simulink model "gm_VSD_and_Park_transformation_6Phase"  (R2022a)
settings: Solver=FixedStepDiscrete  StartTime=0.0  StopTime=0.2  RelTol=1e-3
libraries: hdlmdlgenlib x2
(part 1 of 2)
settings Model: Creator=Andre Merx  LastModifiedBy=Andre Merx
settings SolverCC: AlgebraicLoopSolver=TrustRegion
settings DataIOCC: LimitDataPoints=on  SaveOutput=off  SaveTime=off
settings OptimizationCC: BlockReduction=off  ConditionallyExecuteInputs=off  DefaultParameterBehavior=Inlined  InheritOutputTypeSmallerThanSingle=on  LifeSpan=inf
settings DebuggingCC: AlgebraicLoopMsg=error  InheritedTsInSrcMsg=none  SingleTaskRateTransMsg=error  UnconnectedInputMsg=warning  UnconnectedOutputMsg=warning  UnconnectedLineMsg=warning  AllowSymbolicDim=off  StrictBusMsg=ErrorOnBusTreatedAsVector  SFUnexpectedBacktrackingDiag=warning  SFNoUnconditionalDefaultTransitionDiag=warning  SFExecutionAtInitializationDiag=none  SFMachineParentedDataDiag=warning  ArithmeticOperatorsInVariantConditions=warning
settings HardwareCC: ProdBitPerPointer=32  ProdBitPerSizeT=32  ProdBitPerPtrDiffT=32  ProdLargestAtomicFloat=None  ProdIntDivRoundTo=Undefined  ProdEndianess=Unspecified  ProdWordSize=32  ProdHWDeviceType=ASIC/FPGA->ASIC/FPGA  ProdEqTarget=off
settings SFSimCC: SimUseLocalCustomCode=off  CustomCodeUndefinedFunction=UseInterfaceOnly
settings RTWCC: RTWUseLocalCustomCode=off
settings CodeAppCC: StateflowObjectComments=on
settings GRTTargetCC: TargetLangStandard=C89/C90 (ANSI)
settings ConfigComp: CovScope=ReferencedModels  CovMetricSettings=dw  CovSaveCumulativeToWorkspaceVar=on  CovSaveSingleToWorkspaceVar=on  CovExternalEMLEnable=off  CovSFcnEnable=off

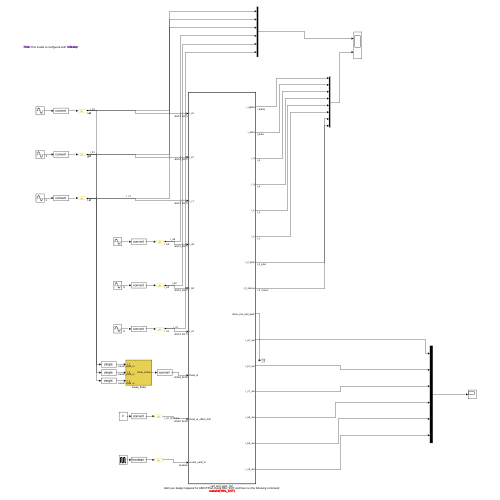
[thumbnail: Simulink's stored preview of the top-level diagram]
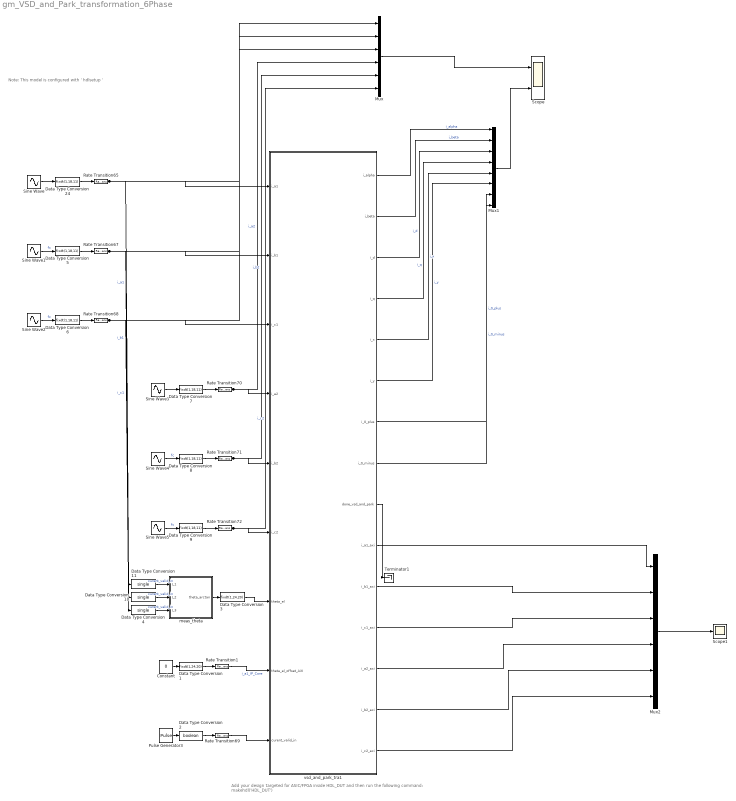
== system gm_VSD_and_Park_transformation_6Phase ==
  note: Add your design targeted for ASIC/FPGA inside HDL_DUT and then run the following command:
      | makehdl('HDL_DUT')
  note: Note: This model is configured with ' hdlsetup '
  Constant : Constant  Value=0  SampleTime=-1
  Data Type Conversion1 : DataTypeConversion  OutDataTypeStr=fixdt(1,24,20)  SaturateOnIntegerOverflow=off  RndMeth=Floor
  Data Type Conversion10 : DataTypeConversion  OutDataTypeStr=single  SaturateOnIntegerOverflow=off  RndMeth=Floor
  Data Type Conversion11 : DataTypeConversion  OutDataTypeStr=single  SaturateOnIntegerOverflow=off  RndMeth=Floor
  Data Type Conversion2 : DataTypeConversion  OutDataTypeStr=boolean  SaturateOnIntegerOverflow=off  RndMeth=Floor
  Data Type Conversion{5..9,24} (6 alike) : DataTypeConversion  OutDataTypeStr=fixdt(1,18,11)  SaturateOnIntegerOverflow=off  RndMeth=Floor
  Data Type Conversion3 : DataTypeConversion  OutDataTypeStr=fixdt(1,24,20)  SaturateOnIntegerOverflow=off  RndMeth=Floor
  Data Type Conversion4 : DataTypeConversion  OutDataTypeStr=single  SaturateOnIntegerOverflow=off  RndMeth=Floor
  Mux : Mux  Inputs=6
  Mux1 : Mux  Inputs=8
  Mux2 : Mux  Inputs=6
  Pulse Generator3 : DiscretePulseGenerator  PulseType=Time based  Period=1/100000  PulseWidth=5
  Rate Transition{1,65,67..72} (8 alike) : RateTransition  OutPortSampleTime=1.0000e-08
  Scope : Scope  NumInputPorts=2
  Scope1 : Scope
  Sine Wave : Sin  Frequency=100  SampleTime=1/100000
  Sine Wave1 : Sin  Frequency=100  Phase=(4/3)*pi  SampleTime=1/100000
  Sine Wave2 : Sin  Frequency=100  Phase=(2/3)*pi  SampleTime=1/100000
  Sine Wave3 : Sin  Amplitude=0.5  Frequency=100  Phase=-pi/6  SampleTime=1/100000
  Sine Wave4 : Sin  Amplitude=0.5  Frequency=100  Phase=(7/6)*pi  SampleTime=1/100000
  Sine Wave5 : Sin  Amplitude=0.5  Frequency=100  Phase=(1/2)*pi  SampleTime=1/100000
  Terminator1 : Terminator
  meas_theta : Subsystem
  vsd_and_park_tra1 : Subsystem  TreatAsAtomicUnit=on
  wires:
  vsd_and_park_tra1/6(i_y) -> Mux1/6  "i_y"
  vsd_and_park_tra1/7(i_0_plus) -> Mux1/7  "i_0_plus"
  vsd_and_park_tra1/8(i_0_minus) -> Mux1/8  "i_0_minus"
  vsd_and_park_tra1/9(done_vsd_and_park) -> Terminator1/1
  Mux2/1 -> Scope1/1
  vsd_and_park_tra1/15(i_c2_axi) -> Mux2/6
  vsd_and_park_tra1/14(i_b2_axi) -> Mux2/5
  vsd_and_park_tra1/13(i_a2_axi) -> Mux2/4
  vsd_and_park_tra1/12(i_c1_axi) -> Mux2/3
  vsd_and_park_tra1/11(i_b1_axi) -> Mux2/2
  vsd_and_park_tra1/10(i_a1_axi) -> Mux2/1
  Data Type Conversion11/1 -> meas_theta/1(I_1)  "curent_valid_in"
  Data Type Conversion10/1 -> meas_theta/2(I_2)  "curent_valid_in"
  Data Type Conversion4/1 -> meas_theta/3(I_3)  "curent_valid_in"
  Data Type Conversion3/1 -> vsd_and_park_tra1/7(theta_el)
  Mux1/1 -> Scope/2
  vsd_and_park_tra1/5(i_x) -> Mux1/5  "i_x"
  vsd_and_park_tra1/4(i_q) -> Mux1/4  "i_q"
  vsd_and_park_tra1/3(i_d) -> Mux1/3  "i_d"
  vsd_and_park_tra1/2(i_beta) -> Mux1/2  "i_beta"
  vsd_and_park_tra1/1(i_alpha) -> Mux1/1  "i_alpha"
  Mux/1 -> Scope/1
  Data Type Conversion2/1 -> Rate Transition69/1
  Rate Transition69/1 -> vsd_and_park_tra1/9(curent_valid_in)
  Pulse Generator3/1 -> Data Type Conversion2/1
  Rate Transition1/1 -> vsd_and_park_tra1/8(theta_el_offset_AXI)  "i_a1_IP_Core"
  Data Type Conversion1/1 -> Rate Transition1/1
  Constant/1 -> Data Type Conversion1/1
  meas_theta/1(theta_arctan) -> Data Type Conversion3/1
  Rate Transition72/1 -> Mux/6, vsd_and_park_tra1/6(i_c2)  "i_c2"
  Rate Transition71/1 -> Mux/5, vsd_and_park_tra1/5(i_b2)  "i_b2"
  Rate Transition70/1 -> Mux/4, vsd_and_park_tra1/4(i_a2)  "i_a2"
  Data Type Conversion8/1 -> Rate Transition71/1
  Data Type Conversion7/1 -> Rate Transition70/1
  Sine Wave3/1 -> Data Type Conversion7/1
  Sine Wave4/1 -> Data Type Conversion8/1  "fc"
  Data Type Conversion9/1 -> Rate Transition72/1
  Sine Wave5/1 -> Data Type Conversion9/1  "fc"
  Rate Transition68/1 -> Mux/3, vsd_and_park_tra1/3(i_c1), Data Type Conversion4/1  "i_c1"
  Rate Transition67/1 -> Data Type Conversion10/1, Mux/2, vsd_and_park_tra1/2(i_b1)  "i_b1"
  Rate Transition65/1 -> Data Type Conversion11/1, Mux/1, vsd_and_park_tra1/1(i_a1)  "i_a1"
  Data Type Conversion24/1 -> Rate Transition65/1
  Data Type Conversion5/1 -> Rate Transition67/1
  Sine Wave2/1 -> Data Type Conversion6/1  "fc"
  Data Type Conversion6/1 -> Rate Transition68/1
  Sine Wave1/1 -> Data Type Conversion5/1  "fc"
  Sine Wave/1 -> Data Type Conversion24/1

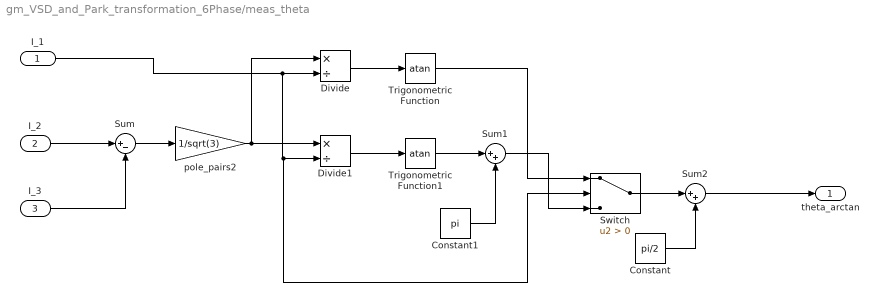
== system gm_VSD_and_Park_transformation_6Phase/meas_theta ==
  I_1 : Inport
  I_2 : Inport  Port=2
  I_3 : Inport  Port=3
  Constant : Constant  Value=pi/2
  Constant1 : Constant  Value=pi
  Divide : Product  Inputs=*/
  Divide1 : Product  Inputs=*/
  Sum : Sum  Inputs=|+-
  Sum1 : Sum  Inputs=|++
  Sum2 : Sum  Inputs=|++
  Switch : Switch  Criteria=u2 > Threshold  SaturateOnIntegerOverflow=off  InputSameDT=off
  Trigonometric Function : Trigonometry  Operator=atan
  Trigonometric Function1 : Trigonometry  Operator=atan
  pole_pairs2 : Gain  Gain=1/sqrt(3)
  theta_arctan : Outport  VectorParamsAs1DForOutWhenUnconnected=off
  wires:
  Sum2/1 -> theta_arctan/1
  Constant1/1 -> Sum1/2
  Constant/1 -> Sum2/2
  Switch/1 -> Sum2/1
  Trigonometric Function/1 -> Switch/1
  Sum1/1 -> Switch/3
  I_1/1 -> Divide/2, Divide1/2, Switch/2
  I_2/1 -> Sum/1
  I_3/1 -> Sum/2
  Sum/1 -> pole_pairs2/1
  pole_pairs2/1 -> Divide1/1, Divide/1
  Trigonometric Function1/1 -> Sum1/1
  Divide1/1 -> Trigonometric Function1/1
  Divide/1 -> Trigonometric Function/1

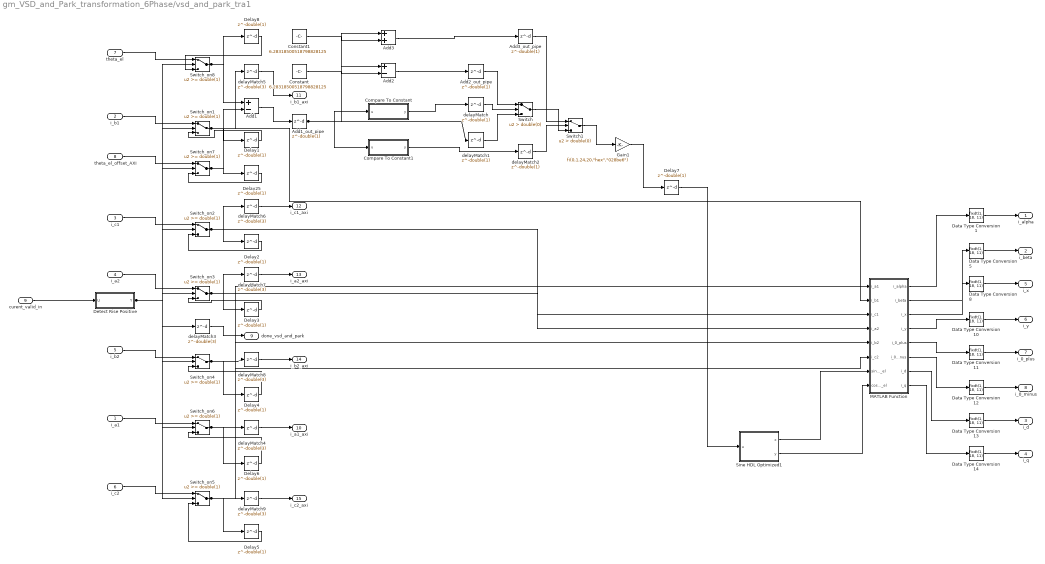
== system gm_VSD_and_Park_transformation_6Phase/vsd_and_park_tra1 ==
  i_a1 : Inport  OutDataTypeStr=fixdt(1, 18, 11)  PortDimensions=1  SampleTime=1e-08
  i_b1 : Inport  Port=2  OutDataTypeStr=fixdt(1, 18, 11)  PortDimensions=1  SampleTime=1e-08
  i_c1 : Inport  Port=3  OutDataTypeStr=fixdt(1, 18, 11)  PortDimensions=1  SampleTime=1e-08
  i_a2 : Inport  Port=4  OutDataTypeStr=fixdt(1, 18, 11)  PortDimensions=1  SampleTime=1e-08
  i_b2 : Inport  Port=5  OutDataTypeStr=fixdt(1, 18, 11)  PortDimensions=1  SampleTime=1e-08
  i_c2 : Inport  Port=6  OutDataTypeStr=fixdt(1, 18, 11)  PortDimensions=1  SampleTime=1e-08
  theta_el : Inport  Port=7  OutDataTypeStr=fixdt(1, 24, 20)  PortDimensions=1  SampleTime=1e-08
  theta_el_offset_AXI : Inport  Port=8  OutDataTypeStr=fixdt(1, 24, 20)  PortDimensions=1  SampleTime=1e-08
  curent_valid_in : Inport  Port=9  OutDataTypeStr=boolean  PortDimensions=1  SampleTime=1e-08
  Add1 : Sum  Inputs=+-  AccumDataTypeStr=fixdt(1, 24, 20)  OutDataTypeStr=fixdt(1, 24, 20)  RndMeth=Simplest  SampleTime=1e-08
  Add1_out_pipe : Delay  DelayLength=double(1)  InitialCondition=0  SampleTime=1e-08
  Add2 : Sum  Inputs=+-  AccumDataTypeStr=fixdt(1, 24, 20)  OutDataTypeStr=fixdt(1, 24, 20)  RndMeth=Simplest  SampleTime=1e-08
  Add2_out_pipe : Delay  DelayLength=double(1)  InitialCondition=0  SampleTime=1e-08
  Add3 : Sum  AccumDataTypeStr=fixdt(1, 24, 20)  OutDataTypeStr=fixdt(1, 24, 20)  RndMeth=Simplest  SampleTime=1e-08
  Add3_out_pipe : Delay  DelayLength=double(1)  InitialCondition=0  SampleTime=1e-08
  Compare To Constant : Subsystem  mask(Compare To Constant){relop=>=, const=double(6.283185307179586), OutDataTypeStr=boolean, ZeroCross=on}
      mask prompts: relop "Simulink:masks:Operator_MP"; const "Simulink:masks:ConstantValue_MP"; OutDataTypeStr "Simulink:masks:OutputDataType_MP"; ZeroCross "Simulink:masks:EnableZerocrossingDetection_MP"
      mask help: Simulink:masks:CompareToConstant_MD
      mask init:
      | OutDataTypeStr = 'boolean';
      | ZeroCross = 'on';
      | blkName = 'VSD_and_Park_transformation_6Phase/vsd_and_park_tra1/Compare\nTo Constant';
      | const = double(6.283185307179586);
      | const_str = '2*pi';
      | const_val = double(6.283185307179586);
      | relop = '>=';
      | setValue = 'boolean';
      | str = '>= 6.2832';
      mask TypeOptions relop: == | ~= | < | <= | >= | >
      mask TypeOptions OutDataTypeStr: Simulink:masks:uint8 | Simulink:masks:boolean
      mask Callback ZeroCross: sl('zeroCrossEnable', gcbh);
      mask Display: disp(str)
  Compare To Constant1 : Subsystem  mask(Compare To Constant){relop=<, const=double(0), OutDataTypeStr=boolean, ZeroCross=on}
      mask prompts: relop "Simulink:masks:Operator_MP"; const "Simulink:masks:ConstantValue_MP"; OutDataTypeStr "Simulink:masks:OutputDataType_MP"; ZeroCross "Simulink:masks:EnableZerocrossingDetection_MP"
      mask help: Simulink:masks:CompareToConstant_MD
      mask init:
      | OutDataTypeStr = 'boolean';
      | ZeroCross = 'on';
      | blkName = 'VSD_and_Park_transformation_6Phase/vsd_and_park_tra1/Compare\nTo Constant1';
      | const = double(0);
      | const_str = '0';
      | const_val = double(0);
      | relop = '<';
      | setValue = 'boolean';
      | str = '< 0';
      mask TypeOptions relop: == | ~= | < | <= | >= | >
      mask TypeOptions OutDataTypeStr: Simulink:masks:uint8 | Simulink:masks:boolean
      mask Callback ZeroCross: sl('zeroCrossEnable', gcbh);
      mask Display: disp(str)
  Constant : Constant  Value=6.28318500518798828125  OutDataTypeStr=fixdt(1, 24, 20)  SampleTime=1e-08
  Constant1 : Constant  Value=6.28318500518798828125  OutDataTypeStr=fixdt(1, 24, 20)  SampleTime=1e-08
  Data Type Conversion{1,5,8,10..14} (8 alike) : DataTypeConversion  OutDataTypeStr=fixdt(1, 18, 11)  SampleTime=1e-08  SaturateOnIntegerOverflow=off  RndMeth=Floor
  Delay{1..8,25} (9 alike) : Delay  DelayLength=double(1)  InitialCondition=0  SampleTime=1e-08
  Detect Rise Positive : Subsystem  mask(Detect Rise Positive){vinit=double(0), InputProcessing=Elements as channels (sample based), OutDataTypeStr=boolean}
      mask prompts: vinit "Simulink:masks:InitialCondition_MP"; InputProcessing "Simulink:masks:InputProcessing_MP"; OutDataTypeStr "Simulink:masks:OutputDataType_MP"
      mask help: Simulink:masks:DetectRisePositive_MD
      mask init:
      | InputProcessing = 'Elements as channels (sample based)';
      | OutDataTypeStr = 'boolean';
      | vinit = double(0);
      mask TypeOptions InputProcessing: Simulink:masks:ColumnsAsChannelsFrameBased | Simulink:masks:ElementsAsChannelsSampleBased
      mask TypeOptions OutDataTypeStr: Simulink:masks:uint8 | Simulink:masks:boolean
      mask Display: fprintf('U > 0\n&  NOT\nU/z > 0')
  Gain1 : Gain  Gain="fi(0,1,24,20,\"hex\",\"028be6\")"  ParamDataTypeStr=fixdt(1, 24, 20)  OutDataTypeStr=fixdt(1, 24, 20)  SampleTime=1e-08
  MATLAB Function : Subsystem
  Sine HDL Optimized1 : Subsystem  mask(Sine and Cosine HDL optimized block){OutputFormula=sin(2*pi*u) and cos(2*pi*u), NumDataPoints=double(512), TableDataTypeStr=fixdt(1,15,14), SimulateLUTROMDelay=off}
      mask prompts: OutputFormula "Simulink:masks:OutputFormula_MP"; NumDataPoints "HDLShared:hdlshared:CosineHDL_Npts"; TableDataTypeStr "Simulink:blkprm_prompts:TABLE_UNIFIEDDATATYPE"; SimulateLUTROMDelay "HDLShared:hdlshared:CosineHDL_SimulateLUTDelay"
      mask help: Sine and Cosine HDL optimized block using quarter wave symmetry, and HDL friendly settings.
      mask Help: helpview([docroot '/hdlcoder/helptargets.map'],'SineAndCosineHDL_Optimized');
      mask TypeOptions OutputFormula: sin(2*pi*u) | cos(2*pi*u) | exp(j*2*pi*u) | sin(2*pi*u) and cos(2*pi*u)
      mask Display:
      | port_label('input',1,'u')
      | port_label('output',1,'sin(2*pi*u)')
      | port_label('output',2,'cos(2*pi*u)')
      | xpos = 0.35;
      | yoffset = 0.5;
      | if ( SimulateLUTROMDelay )
      |   text(xpos,yoffset,'HDL (Z^{-1})','texmode','on')
      | else
      |    text(xpos,yoffset,'HDL')
      | end
  Switch : Switch  Criteria=u2 > Threshold  Threshold=double(0)  OutDataTypeStr=fixdt(1, 24, 20)  RndMeth=Simplest  SampleTime=1e-08  SaturateOnIntegerOverflow=off  InputSameDT=off
  Switch1 : Switch  Criteria=u2 > Threshold  Threshold=double(0)  OutDataTypeStr=fixdt(1, 24, 20)  RndMeth=Simplest  SampleTime=1e-08  SaturateOnIntegerOverflow=off  InputSameDT=off
  Switch_on{1..6} (6 alike) : Switch  Threshold=double(1)  OutDataTypeStr=fixdt(1, 18, 11)  RndMeth=Simplest  SampleTime=1e-08  SaturateOnIntegerOverflow=off  InputSameDT=off
  Switch_on7 : Switch  Threshold=double(1)  OutDataTypeStr=fixdt(1, 24, 20)  RndMeth=Simplest  SampleTime=1e-08  SaturateOnIntegerOverflow=off  InputSameDT=off
  Switch_on8 : Switch  Threshold=double(1)  OutDataTypeStr=fixdt(1, 24, 20)  RndMeth=Simplest  SampleTime=1e-08  SaturateOnIntegerOverflow=off  InputSameDT=off
  delayMatch : Delay  DelayLength=double(1)  InitialCondition=0  SampleTime=1e-08
  delayMatch1 : Delay  DelayLength=double(1)  InitialCondition=0  SampleTime=1e-08
  delayMatch2 : Delay  DelayLength=double(1)  InitialCondition=0  SampleTime=1e-08
  delayMatch{3..9} (7 alike) : Delay  DelayLength=double(3)  InitialCondition=0  SampleTime=1e-08
  i_alpha : Outport  SampleTime=1e-08
  i_beta : Outport  Port=2  SampleTime=1e-08
  i_d : Outport  Port=3  SampleTime=1e-08
  i_q : Outport  Port=4  SampleTime=1e-08
  i_x : Outport  Port=5  SampleTime=1e-08
  i_y : Outport  Port=6  SampleTime=1e-08
  i_0_plus : Outport  Port=7  SampleTime=1e-08
  i_0_minus : Outport  Port=8  SampleTime=1e-08
  done_vsd_and_park : Outport  Port=9  SampleTime=1e-08
  i_a1_axi : Outport  Port=10  SampleTime=1e-08
  i_b1_axi : Outport  Port=11  SampleTime=1e-08
  i_c1_axi : Outport  Port=12  SampleTime=1e-08
  i_a2_axi : Outport  Port=13  SampleTime=1e-08
  i_b2_axi : Outport  Port=14  SampleTime=1e-08
  i_c2_axi : Outport  Port=15  SampleTime=1e-08
  wires:
  i_a1/1 -> Switch_on6/1
  i_b1/1 -> Switch_on1/1
  i_c1/1 -> Switch_on2/1
  i_a2/1 -> Switch_on3/1
  i_b2/1 -> Switch_on4/1
  i_c2/1 -> Switch_on5/1
  theta_el/1 -> Switch_on8/1
  theta_el_offset_AXI/1 -> Switch_on7/1
  curent_valid_in/1 -> Detect Rise Positive/1(U)
  delayMatch1/1 -> Switch/3
  Add2_out_pipe/1 -> Switch/1
  Add3_out_pipe/1 -> Switch1/1
  delayMatch/1 -> Switch/2
  delayMatch2/1 -> Switch1/2
  Constant/1 -> Add2/2
  Constant1/1 -> Add3/2
  Data Type Conversion1/1 -> i_alpha/1
  Data Type Conversion10/1 -> i_y/1
  Data Type Conversion11/1 -> i_0_plus/1
  Data Type Conversion12/1 -> i_0_minus/1
  Data Type Conversion13/1 -> i_d/1
  Data Type Conversion14/1 -> i_q/1
  Data Type Conversion5/1 -> i_beta/1
  Data Type Conversion8/1 -> i_x/1
  Delay7/1 -> Sine HDL Optimized1/1(u)
  delayMatch3/1 -> done_vsd_and_park/1
  Gain1/1 -> Delay7/1
  MATLAB Function/1(i_alpha) -> Data Type Conversion1/1
  MATLAB Function/2(i_beta) -> Data Type Conversion5/1
  MATLAB Function/3(i_x) -> Data Type Conversion8/1
  MATLAB Function/4(i_y) -> Data Type Conversion10/1
  MATLAB Function/5(i_0_plus) -> Data Type Conversion11/1
  MATLAB Function/6(i_0_minus) -> Data Type Conversion12/1
  MATLAB Function/7(i_d) -> Data Type Conversion13/1
  MATLAB Function/8(i_q) -> Data Type Conversion14/1
  Sine HDL Optimized1/1(x) -> MATLAB Function/7(sin_theta_el)
  Sine HDL Optimized1/2(y) -> MATLAB Function/8(cos_theta_el)
  Switch/1 -> Switch1/3
  Switch1/1 -> Gain1/1
  delayMatch5/1 -> i_b1_axi/1
  delayMatch6/1 -> i_c1_axi/1
  delayMatch7/1 -> i_a2_axi/1
  delayMatch8/1 -> i_b2_axi/1
  delayMatch9/1 -> i_c2_axi/1
  delayMatch4/1 -> i_a1_axi/1
  Switch_on7/1 -> Add1/2, Delay25/1
  Switch_on8/1 -> Add1/1, Delay8/1
  Add1/1 -> Add1_out_pipe/1
  Add2/1 -> Add2_out_pipe/1
  Add3/1 -> Add3_out_pipe/1
  Compare To Constant/1(y) -> delayMatch/1
  Add1_out_pipe/1 -> delayMatch1/1, Add3/1, Add2/1, Compare To Constant1/1(u), Compare To Constant/1(u)
  Compare To Constant1/1(y) -> delayMatch2/1
  Detect Rise Positive/1(Y) -> delayMatch3/1, Switch_on6/2, Switch_on1/2, Switch_on2/2, Switch_on3/2, Switch_on4/2, Switch_on5/2, Switch_on8/2, Switch_on7/2
  Switch_on6/1 -> delayMatch4/1, MATLAB Function/1(i_a1), Delay6/1
  Switch_on1/1 -> delayMatch5/1, MATLAB Function/2(i_b1), Delay1/1
  Switch_on2/1 -> delayMatch6/1, MATLAB Function/3(i_c1), Delay2/1
  Switch_on3/1 -> delayMatch7/1, MATLAB Function/4(i_a2), Delay3/1
  Switch_on4/1 -> delayMatch8/1, MATLAB Function/5(i_b2), Delay4/1
  Switch_on5/1 -> delayMatch9/1, MATLAB Function/6(i_c2), Delay5/1
  Delay6/1 -> Switch_on6/3
  Delay1/1 -> Switch_on1/3
  Delay2/1 -> Switch_on2/3
  Delay3/1 -> Switch_on3/3
  Delay4/1 -> Switch_on4/3
  Delay5/1 -> Switch_on5/3
  Delay8/1 -> Switch_on8/3
  Delay25/1 -> Switch_on7/3

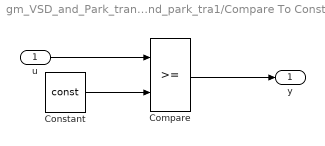
== system gm_VSD_and_Park_transformation_6Phase/vsd_and_park_tra1/Compare To Constant ==
  u : Inport  OutDataTypeStr=fixdt(1, 24, 20)  SampleTime=1e-08
  Compare : RelationalOperator  OutDataTypeStr=boolean
  Constant : Constant  DisableCoverage=on  Value=const  OutDataTypeStr=Inherit: Inherit via back propagation  SampleTime=-1
  y : Outport  SampleTime=1e-08
  wires:
  Compare/1 -> y/1
  Constant/1 -> Compare/2
  u/1 -> Compare/1

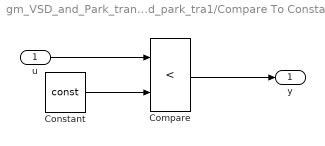
== system gm_VSD_and_Park_transformation_6Phase/vsd_and_park_tra1/Compare To Constant1 ==
  u : Inport  OutDataTypeStr=fixdt(1, 24, 20)  SampleTime=1e-08
  Compare : RelationalOperator  Operator=<  OutDataTypeStr=boolean
  Constant : Constant  DisableCoverage=on  Value=const  OutDataTypeStr=Inherit: Inherit via back propagation  SampleTime=-1
  y : Outport  SampleTime=1e-08
  wires:
  Compare/1 -> y/1
  Constant/1 -> Compare/2
  u/1 -> Compare/1

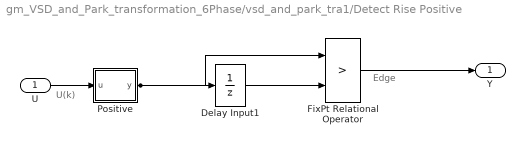
== system gm_VSD_and_Park_transformation_6Phase/vsd_and_park_tra1/Detect Rise Positive ==
  note: Edge
  note: U(k)
  U : Inport  OutDataTypeStr=boolean  SampleTime=1e-08
  Delay Input1 : UnitDelay  Description=Store in Global RAM  DisableCoverage=on  InitialCondition=vinit  SampleTime=-1  HasFrameUpgradeWarning=on
  FixPt Relational Operator : RelationalOperator  Operator=>  OutDataTypeStr=boolean  ZeroCross=off  InputSameDT=off
  Positive : Subsystem  mask(Compare To Zero){relop=>, OutDataTypeStr=boolean, ZeroCross=off}
      mask prompts: relop "Simulink:masks:Operator_MP"; OutDataTypeStr "Simulink:masks:OutputDataType_MP"; ZeroCross "Simulink:masks:EnableZerocrossingDetection_MP"
      mask help: Simulink:masks:CompareToZero_MD
      mask init:
      | OutDataTypeStr = 'boolean';
      | ZeroCross = 'off';
      | blkName = 'VSD_and_Park_transformation_6Phase/vsd_and_park_tra1/Detect Rise\nPositive/Positive';
      | relop = '>';
      | setValue = 'boolean';
      mask TypeOptions relop: == | ~= | < | <= | >= | >
      mask TypeOptions OutDataTypeStr: Simulink:masks:uint8 | Simulink:masks:boolean
      mask Callback ZeroCross: sl('zeroCrossEnable', gcbh);
      mask Display: disp([relop,' 0'])
  Y : Outport  SampleTime=1e-08
  wires:
  Delay Input1/1 -> FixPt Relational Operator/2
  FixPt Relational Operator/1 -> Y/1
  Positive/1(y) -> FixPt Relational Operator/1, Delay Input1/1
  U/1 -> Positive/1(u)

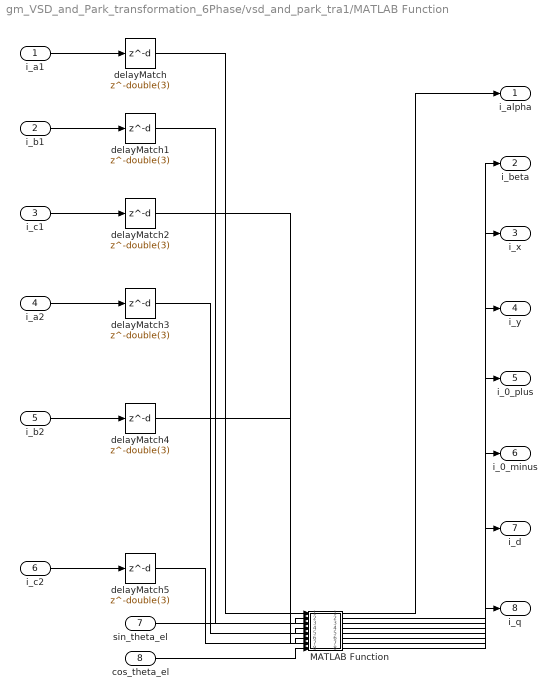
== system gm_VSD_and_Park_transformation_6Phase/vsd_and_park_tra1/MATLAB Function ==
  i_a1 : Inport  OutDataTypeStr=fixdt(1, 18, 11)  PortDimensions=1  SampleTime=1e-08
  i_b1 : Inport  Port=2  OutDataTypeStr=fixdt(1, 18, 11)  PortDimensions=1  SampleTime=1e-08
  i_c1 : Inport  Port=3  OutDataTypeStr=fixdt(1, 18, 11)  PortDimensions=1  SampleTime=1e-08
  i_a2 : Inport  Port=4  OutDataTypeStr=fixdt(1, 18, 11)  PortDimensions=1  SampleTime=1e-08
  i_b2 : Inport  Port=5  OutDataTypeStr=fixdt(1, 18, 11)  PortDimensions=1  SampleTime=1e-08
  i_c2 : Inport  Port=6  OutDataTypeStr=fixdt(1, 18, 11)  PortDimensions=1  SampleTime=1e-08
  sin_theta_el : Inport  Port=7  OutDataTypeStr=fixdt(1, 16, 14)  PortDimensions=1  SampleTime=1e-08
  cos_theta_el : Inport  Port=8  OutDataTypeStr=fixdt(1, 16, 14)  PortDimensions=1  SampleTime=1e-08
  MATLAB Function : MATLAB Function  TreatAsAtomicUnit=on  SystemSampleTime=1/100000000
  delayMatch{,1..5} (6 alike) : Delay  DelayLength=double(3)  InitialCondition=0  SampleTime=1e-08
  i_alpha : Outport  SampleTime=1e-08  VectorParamsAs1DForOutWhenUnconnected=off
  i_beta : Outport  Port=2  SampleTime=1e-08
  i_x : Outport  Port=3  SampleTime=1e-08
  i_y : Outport  Port=4  SampleTime=1e-08
  i_0_plus : Outport  Port=5  SampleTime=1e-08
  i_0_minus : Outport  Port=6  SampleTime=1e-08
  i_d : Outport  Port=7  SampleTime=1e-08
  i_q : Outport  Port=8  SampleTime=1e-08
  wires:
  delayMatch/1 -> MATLAB Function/1(i_a1)
  delayMatch1/1 -> MATLAB Function/2(i_b1)
  delayMatch2/1 -> MATLAB Function/3(i_c1)
  delayMatch3/1 -> MATLAB Function/4(i_a2)
  delayMatch4/1 -> MATLAB Function/5(i_b2)
  delayMatch5/1 -> MATLAB Function/6(i_c2)
  MATLAB Function/1(i_alpha) -> i_alpha/1
  MATLAB Function/2(i_beta) -> i_beta/1
  MATLAB Function/3(i_x) -> i_x/1
  MATLAB Function/4(i_y) -> i_y/1
  MATLAB Function/5(i_0_plus) -> i_0_plus/1
  MATLAB Function/6(i_0_minus) -> i_0_minus/1
  MATLAB Function/7(i_d) -> i_d/1
  MATLAB Function/8(i_q) -> i_q/1
  i_a1/1 -> delayMatch/1
  i_b1/1 -> delayMatch1/1
  i_c1/1 -> delayMatch2/1
  i_a2/1 -> delayMatch3/1
  i_b2/1 -> delayMatch4/1
  i_c2/1 -> delayMatch5/1
  sin_theta_el/1 -> MATLAB Function/7(sin_theta_el)
  cos_theta_el/1 -> MATLAB Function/8(cos_theta_el)

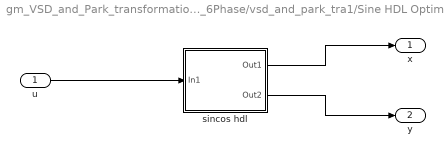
== system gm_VSD_and_Park_transformation_6Phase/vsd_and_park_tra1/Sine HDL Optimized1 ==
  u : Inport  OutDataTypeStr=fixdt(1, 24, 20)  SampleTime=1e-08
  sincos hdl : Subsystem  mask{NumDataPoints=512, TableDataTypeStr=fixdt(1,15,14), SimulateLUTROMDelay='Off'}
      mask prompts: NumDataPoints "HDLShared:hdlshared:CosineHDL_Npts"; TableDataTypeStr "Simulink:blkprm_prompts:TABLE_UNIFIEDDATATYPE"; SimulateLUTROMDelay "HDLShared:hdlshared:CosineHDL_SimulateLUTDelay"
      mask Display:
      | port_label('input',1,'u')
      | port_label('output',1,'sin(2*pi*u)')
      | port_label('output',2,'cos(2*pi*u)')
      | xpos = 0.35;
      | yoffset = 0.5;
      | if ( SimulateLUTROMDelay )
      |   text(xpos,yoffset,'HDL (Z^{-1})','texmode','on')
      | else
      |    text(xpos,yoffset,'HDL')
      | end
  x : Outport  SampleTime=1e-08
  y : Outport  Port=2  SampleTime=1e-08
  wires:
  sincos hdl/1(Out1) -> x/1
  sincos hdl/2(Out2) -> y/1
  u/1 -> sincos hdl/1(In1)

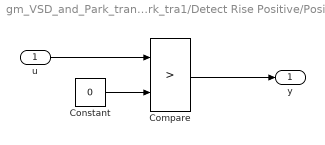
== system gm_VSD_and_Park_transformation_6Phase/vsd_and_park_tra1/Detect Rise Positive/Positive ==
  u : Inport  OutDataTypeStr=boolean  SampleTime=1e-08
  Compare : RelationalOperator  Operator=>  OutDataTypeStr=boolean  ZeroCross=off
  Constant : Constant  DisableCoverage=on  Value=0  OutDataTypeStr=Inherit: Inherit via back propagation  SampleTime=-1  PreserveConstantTs=on
  y : Outport  SampleTime=1e-08
  wires:
  Compare/1 -> y/1
  Constant/1 -> Compare/2
  u/1 -> Compare/1

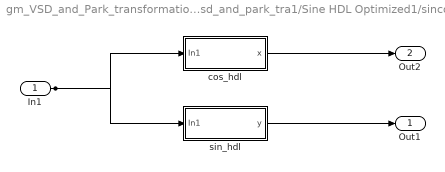
== system gm_VSD_and_Park_transformation_6Phase/vsd_and_park_tra1/Sine HDL Optimized1/sincos hdl ==
  In1 : Inport  OutDataTypeStr=fixdt(1, 24, 20)  SampleTime=1e-08
  cos_hdl : Subsystem  mask{NumDataPoints=double(512), TableDataTypeStr=fixdt(1,15,14), SimulateLUTROMDelay=Off}
      mask prompts: NumDataPoints "HDLShared:hdlshared:CosineHDL_Npts"; TableDataTypeStr "Simulink:blkprm_prompts:TABLE_UNIFIEDDATATYPE"; SimulateLUTROMDelay "HDLShared:hdlshared:CosineHDL_SimulateLUTDelay"
      mask Display:
      | port_label('input',1,'u')
      | port_label('output',1,'cos(2*pi*u)')
      | xpos = 0.35;
      | yoffset = 0.5;
      | if ( SimulateLUTROMDelay )
      |   text(xpos,yoffset,'HDL (Z^{-1})','texmode','on')
      | else
      |    text(xpos,yoffset,'HDL')
      | end
  sin_hdl : Subsystem  mask{NumDataPoints=double(512), TableDataTypeStr=fixdt(1,15,14), SimulateLUTROMDelay=Off}
      mask prompts: NumDataPoints "HDLShared:hdlshared:CosineHDL_Npts"; TableDataTypeStr "Simulink:blkprm_prompts:TABLE_UNIFIEDDATATYPE"; SimulateLUTROMDelay "HDLShared:hdlshared:CosineHDL_SimulateLUTDelay"
      mask Display:
      | port_label('input',1,'u')
      | port_label('output',1,'sin(2*pi*u)')
      | xpos = 0.35;
      | yoffset = 0.5;
      | if ( SimulateLUTROMDelay )
      |   text(xpos,yoffset,'HDL (Z^{-1})','texmode','on')
      | else
      |    text(xpos,yoffset,'HDL')
      | end
  Out1 : Outport  SampleTime=1e-08
  Out2 : Outport  Port=2  SampleTime=1e-08
  wires:
  cos_hdl/1(x) -> Out2/1
  sin_hdl/1(y) -> Out1/1
  In1/1 -> cos_hdl/1(In1), sin_hdl/1(In1)

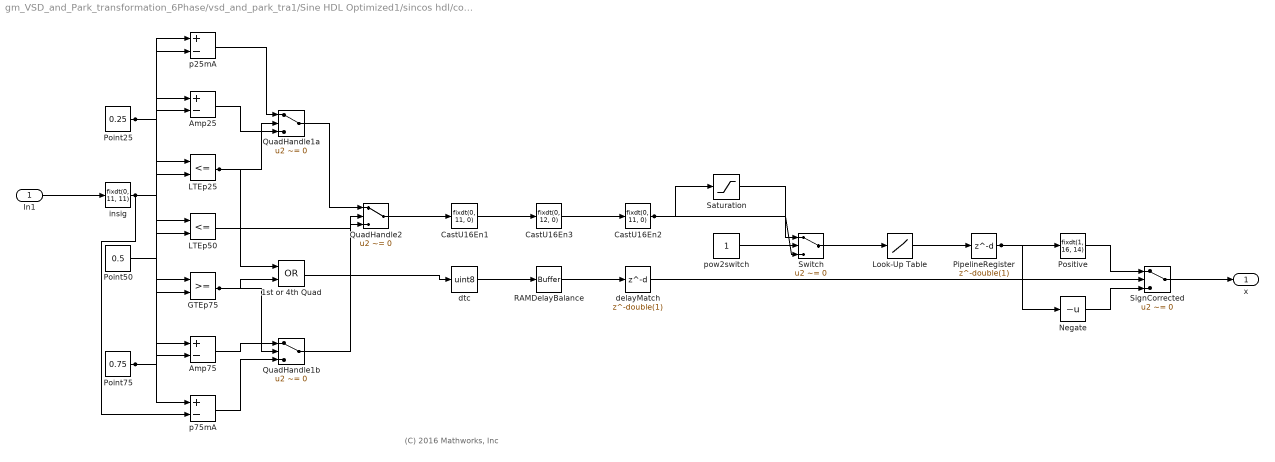
== system gm_VSD_and_Park_transformation_6Phase/vsd_and_park_tra1/Sine HDL Optimized1/sincos hdl/cos_hdl ==
  note: (C) 2016 Mathworks, Inc
  In1 : Inport  OutDataTypeStr=fixdt(1, 24, 20)  SampleTime=1e-08
  1st or 4th Quad : Logic  Operator=OR  AllPortsSameDT=off  OutDataTypeStr=boolean  SampleTime=1e-08
  Amp25 : Sum  Inputs=+-  AccumDataTypeStr=fixdt(1, 17, 16)  OutDataTypeStr=fixdt(1, 17, 16)  SampleTime=1e-08
  Amp75 : Sum  Inputs=+-  AccumDataTypeStr=fixdt(1, 17, 16)  OutDataTypeStr=fixdt(1, 17, 16)  SampleTime=1e-08
  CastU16En1 : DataTypeConversion  OutDataTypeStr=fixdt(0, 11, 0)  ConvertRealWorld=Stored Integer (SI)  SampleTime=1e-08  SaturateOnIntegerOverflow=off  RndMeth=Floor
  CastU16En2 : DataTypeConversion  OutDataTypeStr=fixdt(0, 11, 0)  ConvertRealWorld=Stored Integer (SI)  SampleTime=1e-08  RndMeth=Floor
  CastU16En3 : DataTypeConversion  OutDataTypeStr=fixdt(0, 12, 0)  SampleTime=1e-08  SaturateOnIntegerOverflow=off  RndMeth=Floor
  GTEp75 : RelationalOperator  OutDataTypeStr=boolean  SampleTime=1e-08  InputSameDT=off
  LTEp25 : RelationalOperator  Operator=<=  OutDataTypeStr=boolean  SampleTime=1e-08  InputSameDT=off
  LTEp50 : RelationalOperator  Operator=<=  OutDataTypeStr=boolean  SampleTime=1e-08  InputSameDT=off
  Look-Up Table : Lookup_n-D  NumberOfTableDimensions=1  BreakpointsForDimension1="fi(\"numerictype\",numerictype(0,11,0),\"fimath\",fimath(\"RoundingMethod\", \"Floor\",\"OverflowAction\", \"Wrap\",\"ProductMode\",\"FullPrecision\",\"SumMode\",\"FullPrecision\"),\"Value\",\"[0 1 2 3 4 5 6 7 8 9 10 11 12 13 14 15 16 17 18 19 20 21 22 23 24 25 26 27 28 29 30 31 32 33 34 35 36 37 38 39 40 41 42 43 44 45 46 47 48 49 50 51 52 53 54 55 56 57 58 59 60 61 62 63 64 65 66 67 68 69 70 71 72 73 74 75 76 77 78 79 80 81 82 83 84 85 86 87 88 89 90 91 92 93 94 95 96 97 98 99 100 101 102 103 104 105 106 107 108 109 110 111 112 113 114 115 116 117 118 119 120 121 122 123 124 125 126 127 128 129 130 131 132 133 134 135 136 137 138 139 140 141 142 143 144 145 146 147 148 149 150 151 152 153 154 155 156 157 158 159 160 161 162 163 164 165 166 167 168 169 170 171 172 173 174 175 176 177 178 179 180 181 182 183 184 185 186 187 188 189 190 191 192 193 194 195 196 197 198 199 200 201 202 203 204 205 206 207 208 209 210 211 212 213 214 215 216 217 218 219 220 221 222 223 224 225 226 227 228 229 230 231 232 233 234 235 236 237 238 239 240 241 242 243 244 245 246 247 248 249 250 251 252 253 254 255 256 257 258 259 260 261 262 263 264 265 266 267 268 269 270 271 272 273 274 275 276 277 278 279 280 281 282 283 284 285 286 287 288 289 290 291 292 293 294 295 296 297 298 299 300 301 302 303 304 305 306 307 308 309 310 311 312 313 314 315 316 317 318 319 320 321 322 323 324 325 326 327 328 329 330 331 332 333 334 335 336 337 338 339 340 341 342 343 344 345 346 347 348 349 350 351 352 353 354 355 356 357 358 359 360 361 362 363 364 365 366 367 368 369 370 371 372 373 374 375 376 377 378 379 380 381 382 383 384 385 386 387 388 389 390 391 392 393 394 395 396 397 398 399 400 401 402 403 404 405 406 407 408 409 410 411 412 413 414 415 416 417 418 419 420 421 422 423 424 425 426 427 428 429 430 431 432 433 434 435 436 437 438 439 440 441 442 443 444 445 446 447 448 449 450 451 452 453 454 455 456 457 458 459 460 461 462 463 464 465 466 467 468 469 470 471 472 473 474 475 476 477 478 479 480 481 482 483 484 485 486 487 488 489 490 491 492 493 494 495 496 497 498 499 500 501 502 503 504 505 506 507 508 509 510 511]\")"  Table="reshape(fi(\"numerictype\",numerictype(1,16,14),\"fimath\",fimath(\"RoundingMethod\", \"Floor\",\"OverflowAction\", \"Wrap\",\"ProductMode\",\"FullPrecision\",\"SumMode\",\"FullPrecision\"),\"Value\",\"[0;0.0030517578125;0.00616455078125;0.00921630859375;0.01226806640625;0.015380859375;0.0184326171875;0.02154541015625;0.02459716796875;0.02764892578125;0.03076171875;0.0338134765625;0.036865234375;0.03997802734375;0.04302978515625;0.04608154296875;0.04913330078125;0.05224609375;0.0552978515625;0.058349609375;0.06146240234375;0.06451416015625;0.06756591796875;0.07061767578125;0.07373046875;0.0767822265625;0.079833984375;0.0828857421875;0.0859375;0.08905029296875;0.09210205078125;0.09515380859375;0.09820556640625;0.10125732421875;0.10430908203125;0.10736083984375;0.11041259765625;0.11346435546875;0.11651611328125;0.11956787109375;0.12261962890625;0.12567138671875;0.12872314453125;0.13177490234375;0.13482666015625;0.13787841796875;0.14093017578125;0.14398193359375;0.14703369140625;0.15008544921875;0.153076171875;0.1561279296875;0.1591796875;0.16217041015625;0.16522216796875;0.16827392578125;0.1712646484375;0.17431640625;0.1773681640625;0.18035888671875;0.18341064453125;0.1864013671875;0.189453125;0.19244384765625;0.19549560546875;0.198486328125;0.20147705078125;0.20452880859375;0.20751953125;0.21051025390625;0.2135009765625;0.216552734375;0.21954345703125;0.2225341796875;0.22552490234375;0.228515625;0.23150634765625;0.2344970703125;0.23748779296875;0.240478515625;0.24346923828125;0.24639892578125;0.2493896484375;0.25238037109375;0.25537109375;0.25830078125;0.26129150390625;0.2642822265625;0.2672119140625;0.27020263671875;0.27313232421875;0.276123046875;0.279052734375;0.281982421875;0.28497314453125;0.28790283203125;0.29083251953125;0.29376220703125;0.29669189453125;0.29962158203125;0.30255126953125;0.30548095703125;0.30841064453125;0.31134033203125;0.31427001953125;0.31719970703125;0.32012939453125;0.322998046875;0.325927734375;0.328857421875;0.33172607421875;0.33465576171875;0.3375244140625;0.34039306640625;0.34332275390625;0.34619140625;0.34906005859375;0.3519287109375;0.35479736328125;0.35772705078125;0.360595703125;0.3634033203125;0.36627197265625;0.369140625;0.37200927734375;0.3748779296875;0.377685546875;0.38055419921875;0.3834228515625;0.38623046875;0.3890380859375;0.39190673828125;0.39471435546875;0.39752197265625;0.400390625;0.4031982421875;0.406005859375;0.4088134765625;0.41162109375;0.41436767578125;0.41717529296875;0.41998291015625;0.42279052734375;0.425537109375;0.4283447265625;0.43109130859375;0.43389892578125;0.4366455078125;0.43939208984375;0.44219970703125;0.4449462890625;0.44769287109375;0.450439453125;0.45318603515625;0.4559326171875;0.4586181640625;0.46136474609375;0.464111328125;0.466796875;0.46954345703125;0.47222900390625;0.4749755859375;0.4776611328125;0.4803466796875;0.4830322265625;0.4857177734375;0.4884033203125;0.4910888671875;0.4937744140625;0.4964599609375;0.49908447265625;0.50177001953125;0.50445556640625;0.507080078125;0.50970458984375;0.51239013671875;0.5150146484375;0.51763916015625;0.520263671875;0.52288818359375;0.5255126953125;0.52813720703125;0.53070068359375;0.5333251953125;0.53594970703125;0.53851318359375;0.5411376953125;0.543701171875;0.5462646484375;0.548828125;0.5513916015625;0.553955078125;0.5565185546875;0.55908203125;0.5616455078125;0.56414794921875;0.56671142578125;0.5692138671875;0.57177734375;0.57427978515625;0.5767822265625;0.57928466796875;0.581787109375;0.58428955078125;0.5867919921875;0.58929443359375;0.59173583984375;0.59423828125;0.5966796875;0.59918212890625;0.60162353515625;0.60406494140625;0.60650634765625;0.60894775390625;0.61138916015625;0.61383056640625;0.61627197265625;0.61865234375;0.62109375;0.62347412109375;0.62591552734375;0.6282958984375;0.63067626953125;0.633056640625;0.63543701171875;0.6378173828125;0.64019775390625;0.64251708984375;0.6448974609375;0.647216796875;0.6495361328125;0.65191650390625;0.65423583984375;0.65655517578125;0.65887451171875;0.66119384765625;0.6634521484375;0.665771484375;0.6680908203125;0.67034912109375;0.672607421875;0.6749267578125;0.67718505859375;0.679443359375;0.68170166015625;0.68389892578125;0.6861572265625;0.68841552734375 ...(+4183 chars)]\"), [1  512])"  InterpMethod=Flat  ExtrapMethod=Clip  DiagnosticForOutOfRangeInput=Error  SampleTime=1e-08  OutDataTypeStr=fixdt(1, 16, 14)
  Negate : UnaryMinus  SampleTime=1e-08
  PipelineRegister : Delay  DelayLength=double(1)  InitialCondition=0  SampleTime=1e-08
  Point25 : Constant  Value=0.25  OutDataTypeStr=fixdt(0, 16, 16)  SampleTime=1e-08
  Point50 : Constant  Value=0.5  OutDataTypeStr=fixdt(0, 16, 16)  SampleTime=1e-08
  Point75 : Constant  Value=0.75  OutDataTypeStr=fixdt(0, 16, 16)  SampleTime=1e-08
  Positive : DataTypeConversion  OutDataTypeStr=fixdt(1, 16, 14)  SampleTime=1e-08  SaturateOnIntegerOverflow=off  RndMeth=Floor
  QuadHandle1a : Switch  Criteria=u2 ~= 0  Threshold=double(0)  OutDataTypeStr=fixdt(1, 17, 16)  SampleTime=1e-08  SaturateOnIntegerOverflow=off  InputSameDT=off
  QuadHandle1b : Switch  Criteria=u2 ~= 0  Threshold=double(0)  OutDataTypeStr=fixdt(1, 17, 16)  SampleTime=1e-08  SaturateOnIntegerOverflow=off  InputSameDT=off
  QuadHandle2 : Switch  Criteria=u2 ~= 0  Threshold=double(0)  OutDataTypeStr=fixdt(0, 11, 11)  SampleTime=1e-08  InputSameDT=off
  RAMDelayBalance : hdlmdlgenlib/Buffer
      settings: SourceProductBaseCode=SL
  Saturation : Saturate  UpperLimit="fi(0,0,11,0,\"hex\",\"1ff\")"  LowerLimit="fi(0,0,11,0,\"hex\",\"000\")"  SampleTime=1e-08  OutDataTypeStr=fixdt(0, 11, 0)
  SignCorrected : Switch  Criteria=u2 ~= 0  Threshold=double(0)  OutDataTypeStr=fixdt(1, 16, 14)  SampleTime=1e-08  SaturateOnIntegerOverflow=off  InputSameDT=off
  Switch : Switch  Criteria=u2 ~= 0  Threshold=double(0)  OutDataTypeStr=fixdt(0, 11, 0)  SampleTime=1e-08  SaturateOnIntegerOverflow=off  InputSameDT=off
  delayMatch : Delay  DelayLength=double(1)  InitialCondition=0  SampleTime=1e-08
  dtc : DataTypeConversion  OutDataTypeStr=uint8  SampleTime=1e-08  SaturateOnIntegerOverflow=off  RndMeth=Floor
  insig : DataTypeConversion  OutDataTypeStr=fixdt(0, 11, 11)  SampleTime=1e-08  SaturateOnIntegerOverflow=off  RndMeth=Floor
  p25mA : Sum  Inputs=+-  AccumDataTypeStr=fixdt(1, 17, 16)  OutDataTypeStr=fixdt(1, 17, 16)  SampleTime=1e-08
  p75mA : Sum  Inputs=+-  AccumDataTypeStr=fixdt(1, 17, 16)  OutDataTypeStr=fixdt(1, 17, 16)  SampleTime=1e-08
  pow2switch : Constant  OutDataTypeStr=boolean  SampleTime=1e-08
  x : Outport  SampleTime=1e-08
  wires:
  dtc/1 -> RAMDelayBalance/1
  Amp25/1 -> QuadHandle1a/3
  Amp75/1 -> QuadHandle1b/1
  CastU16En1/1 -> CastU16En3/1
  CastU16En2/1 -> Switch/3, Saturation/1
  CastU16En3/1 -> CastU16En2/1
  GTEp75/1 -> QuadHandle1b/2, 1st or 4th Quad/2
  LTEp25/1 -> QuadHandle1a/2, 1st or 4th Quad/1
  LTEp50/1 -> QuadHandle2/2
  PipelineRegister/1 -> Positive/1, Negate/1
  Negate/1 -> SignCorrected/3
  Point25/1 -> p25mA/1, LTEp25/2, Amp25/2
  Point50/1 -> LTEp50/2
  Point75/1 -> p75mA/1, GTEp75/2, Amp75/2
  Positive/1 -> SignCorrected/1
  QuadHandle1a/1 -> QuadHandle2/1
  QuadHandle1b/1 -> QuadHandle2/3
  QuadHandle2/1 -> CastU16En1/1
  delayMatch/1 -> SignCorrected/2
  Saturation/1 -> Switch/1
  SignCorrected/1 -> x/1
  Switch/1 -> Look-Up Table/1
  insig/1 -> p75mA/2, p25mA/2, LTEp50/1, LTEp25/1, GTEp75/1, Amp75/1, Amp25/1
  p25mA/1 -> QuadHandle1a/1
  p75mA/1 -> QuadHandle1b/3
  pow2switch/1 -> Switch/2
  1st or 4th Quad/1 -> dtc/1
  In1/1 -> insig/1
  RAMDelayBalance/1 -> delayMatch/1
  Look-Up Table/1 -> PipelineRegister/1
